simulink model "gm_Laba2"  (R2022a)
settings: Solver=VariableStepAuto  StartTime=0.0  StopTime=10.0  RelTol=1e-3
settings Model: Creator=38098  LastModifiedBy=38098
settings OptimizationCC: BlockReduction=off  ConditionallyExecuteInputs=off
settings DebuggingCC: InheritedTsInSrcMsg=none

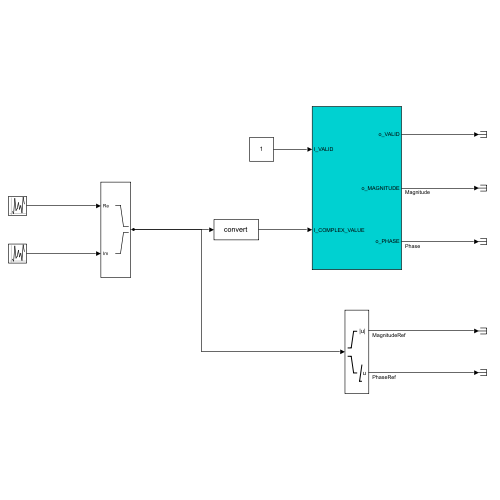
[thumbnail: Simulink's stored preview of the top-level diagram]
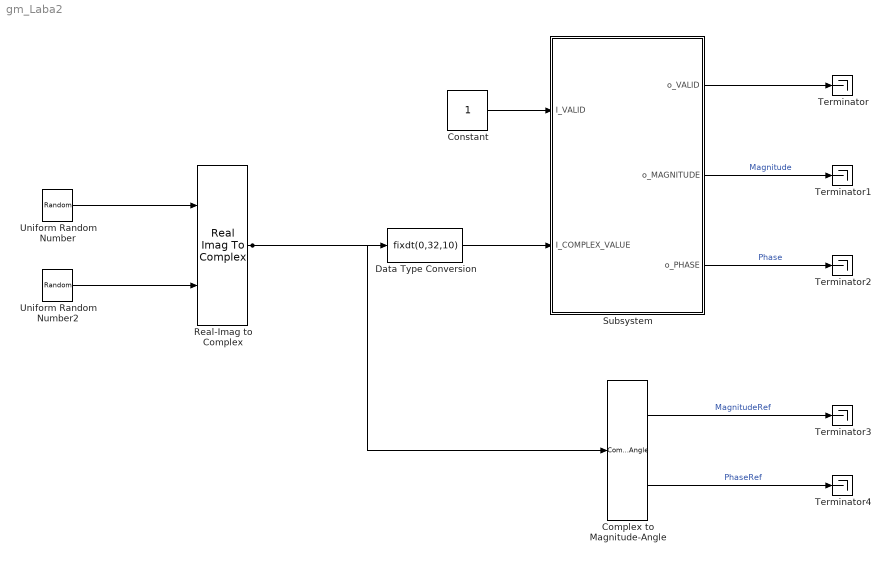
== system gm_Laba2 ==
  Complex to Magnitude-Angle : ComplexToMagnitudeAngle
  Constant : Constant  OutDataTypeStr=boolean
  Data Type Conversion : DataTypeConversion  OutDataTypeStr=fixdt(0,32,10)  RndMeth=Round  SaturateOnIntegerOverflow=off
  Real-Imag to Complex : RealImagToComplex
  Subsystem : Subsystem
  Terminator{,1..4} (5 alike) : Terminator
  Uniform Random Number : UniformRandomNumber  Minimum=0  Maximum=2^(22)-1  Seed=22  SampleTime=1
  Uniform Random Number2 : UniformRandomNumber  Minimum=0  Maximum=2^(22)-1  Seed=23  SampleTime=1
  wires:
  Subsystem/3(o_PHASE) -> Terminator2/1  "Phase"
  Subsystem/2(o_MAGNITUDE) -> Terminator1/1  "Magnitude"
  Subsystem/1(o_VALID) -> Terminator/1
  Data Type Conversion/1 -> Subsystem/2(I_COMPLEX_VALUE)
  Constant/1 -> Subsystem/1(I_VALID)
  Complex to Magnitude-Angle/2 -> Terminator4/1  "PhaseRef"
  Complex to Magnitude-Angle/1 -> Terminator3/1  "MagnitudeRef"
  Real-Imag to Complex/1 -> Data Type Conversion/1, Complex to Magnitude-Angle/1
  Uniform Random Number2/1 -> Real-Imag to Complex/2
  Uniform Random Number/1 -> Real-Imag to Complex/1

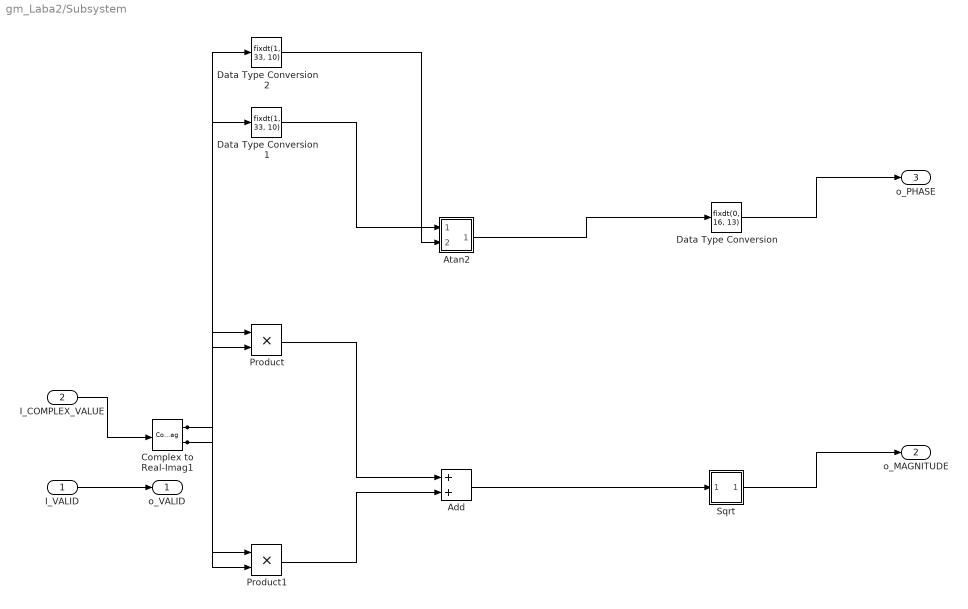
== system gm_Laba2/Subsystem ==
  I_VALID : Inport  OutDataTypeStr=boolean  PortDimensions=1
  I_COMPLEX_VALUE : Inport  Port=2  OutDataTypeStr=fixdt(0, 32, 10)  PortDimensions=1  SampleTime=1
      settings: SignalType=complex
  Add : Sum  AccumDataTypeStr=fixdt(0, 65, 20)  OutDataTypeStr=fixdt(0, 65, 20)  SampleTime=1
  Atan2 : Subsystem
  Complex to Real-Imag1 : ComplexToRealImag  SampleTime=1
  Data Type Conversion : DataTypeConversion  OutDataTypeStr=fixdt(0, 16, 13)  RndMeth=Round  SampleTime=1  SaturateOnIntegerOverflow=off
  Data Type Conversion1 : DataTypeConversion  OutDataTypeStr=fixdt(1, 33, 10)  SampleTime=1  SaturateOnIntegerOverflow=off  RndMeth=Floor
  Data Type Conversion2 : DataTypeConversion  OutDataTypeStr=fixdt(1, 33, 10)  SampleTime=1  SaturateOnIntegerOverflow=off  RndMeth=Floor
  Product : Product  Inputs=**  OutDataTypeStr=fixdt(0, 64, 20)  SampleTime=1
  Product1 : Product  Inputs=**  OutDataTypeStr=fixdt(0, 64, 20)  SampleTime=1
  Sqrt : Subsystem
  o_VALID : Outport
  o_MAGNITUDE : Outport  Port=2  SampleTime=1
  o_PHASE : Outport  Port=3  SampleTime=1
  wires:
  I_VALID/1 -> o_VALID/1
  I_COMPLEX_VALUE/1 -> Complex to Real-Imag1/1
  Add/1 -> Sqrt/1(In1)
  Atan2/1(Out1) -> Data Type Conversion/1
  Complex to Real-Imag1/1 -> Product/2, Product/1, Data Type Conversion2/1
  Complex to Real-Imag1/2 -> Product1/2, Product1/1, Data Type Conversion1/1
  Data Type Conversion/1 -> o_PHASE/1
  Data Type Conversion1/1 -> Atan2/1(In1)
  Data Type Conversion2/1 -> Atan2/2(In2)
  Product/1 -> Add/1
  Product1/1 -> Add/2
  Sqrt/1(Out1) -> o_MAGNITUDE/1

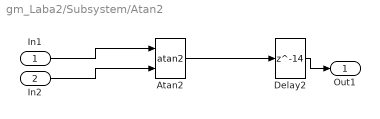
== system gm_Laba2/Subsystem/Atan2 ==
  In1 : Inport
  In2 : Inport  Port=2
  Atan2 : Trigonometry  Operator=atan2  ApproximationMethod=CORDIC
  Delay2 : Delay  DelayLength=14
  Out1 : Outport
  wires:
  In1/1 -> Atan2/1
  In2/1 -> Atan2/2
  Atan2/1 -> Delay2/1
  Delay2/1 -> Out1/1

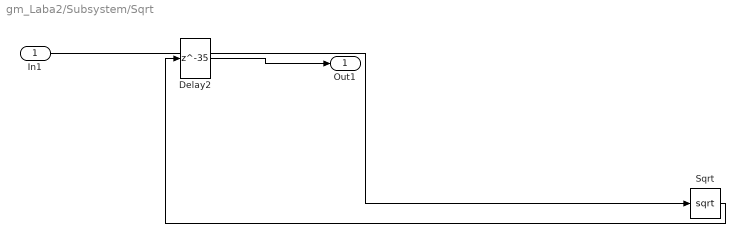
== system gm_Laba2/Subsystem/Sqrt ==
  In1 : Inport
  Delay2 : Delay  DelayLength=35
  Sqrt : Sqrt  OutDataTypeStr=Inherit: Inherit via internal rule
  Out1 : Outport
  wires:
  In1/1 -> Sqrt/1
  Sqrt/1 -> Delay2/1
  Delay2/1 -> Out1/1
